simulink model "PVRobusMPC_final"  (R2018a)
settings: Solver=ode2  StartTime=0.0  StopTime=43200  FixedStep=1  RelTol=1e-3  EnableMultiTasking=on
InitFcn:
  | load PV_model_data
StopFcn:
  | save results Lambda_UV01 T_PV_Reference Tm_f01 Pout01 Tamb Time
  | clear all
  | load results
  | figure
  | subplot(3,1,1)
  | plot(Time./3600,T_PV_Reference,Time./3600,Tm_f01)
  | legend('PV Temperature Reference','PV Temperature')
  | title('MPC Tracking')
  | ylim([350 380])
  | subplot(3,1,2)
  | plot(Time./3600,Lambda_UV01)
  | ylim([250 450])
  | legend('\lambda_U_V')
  | subplot(3,1,3)
  | plot(Time./3600,Pout01)
  | legend('PV Power')
  | xlabel('Time [hours]')
  | ylabel('Watt')
values from neighbouring files (symbols this model uses):
  Global_tilt_Irr_2_2_12_13_5 = [0.000279 0.000786 0.00115 0.00401 0.0047 0.0102 0.011 0.0195 0.0266 0.0299 0.0338 0.0682 ... (2802 elements, 1401x2)]    [PV_model_data.mat]
  Total_light_absorption_in_polystyren = [0.0148235487596 0.0159326919994 0.0170383922491 0.0181406655151 0.0192395277052 0.0203349946285 0.0214270819969 0.0225158054254 0.0236011804327 0.0246832224425 0.0257619467839 0.0264640052027 ... (1151 elements, 1151x1)]    [PV_model_data.mat]
  Total_light_absorption_in_PV_cell_acrylic = [0.0222539070262 0.0239185757929 0.0255780524095 0.0272323791236 0.0288816001883 0.030525761736 0.0321649116541 0.0337990994657 0.0354283762117 0.0370527943369 0.0386724075795 0.0397267002838 ... (1151 elements, 1151x1)]    [PV_model_data.mat]
libraries: mpclib x256
(part 14 of 72)

== system PVRobusMPC_final/4 x 4 x 4 PV Panel 2/4 x 4 PV Panel 8/4 PV Panel 2/PV Panel 8/Photovolatic Panel ==
  Lambda_UV : Inport
  Lambda_IR : Inport  Port=2
  Tambient : Inport  Port=3
  WS : Inport  Port=4
  PV_Cell_Model : MATLAB Function  TreatAsAtomicUnit=on
  Step Size [sec] : Constant
  Unit Delay : UnitDelay  InitialCondition=Temp_Initial  SampleTime=-1
  Tm_f [K] : Outport
  Pout [Watt] : Outport  Port=2
  Vout [Volts] : Outport  Port=3
  wires:
  WS/1 -> PV_Cell_Model/6(WS)
  Tambient/1 -> PV_Cell_Model/5(Tambient)
  PV_Cell_Model/2(QQ) -> Pout [Watt]/1
  Unit Delay/1 -> PV_Cell_Model/1(Tm_i)
  PV_Cell_Model/1(Tm_f) -> Unit Delay/1, Tm_f [K]/1
  Lambda_UV/1 -> PV_Cell_Model/2(Lambda_UV)
  Lambda_IR/1 -> PV_Cell_Model/3(Lambda_IR)
  Step Size [sec]/1 -> PV_Cell_Model/4(Time)
  PV_Cell_Model/3(VL) -> Vout [Volts]/1

== system PVRobusMPC_final/4 x 4 x 4 PV Panel 2/4 x 4 PV Panel 8/4 PV Panel 3/PV Panel 5/PV MPC ==
  Tm_f : Inport
  Tambient : Inport  Port=2
  Fcn : Fcn  Expr=0.916 *u(1)+79
  MPC Controller : mpclib/MPC Controller  SCDEnableBlockLinearizationSpecification=on  mpcobj=mpc1  is_multiple=0  enable_value=0  return_u0=off  updateMPCinCallerWorkspace=on  ref_from_ws=off  ref_signal_name=[]  ref_preview=off  md_from_ws=off  md_signal_name=[]  md_preview=off  from_project=off  project_file=MPCtask.mat  md_inport=off  mv_inport=off  cost_outport=off  return_sequence=off  return_qpstatus=off  return_state=off  state_inport=off  lims_inport=off  cc_inport=off  ywt_inport=off  is_designfromscratch=0  uwt_inport=off  duwt_inport=off  rhoeps_inport=off  uref_inport=off  n_ts=10  n_p=10  n_mv=1  n_md=1  n_ud=0  n_mo=1  n_uo=0  BlockDataType=double  SampleTimeInherited=off  switch_inport=off
  Rate Transition1 : RateTransition  OutPortSampleTime=1
  Rate Transition2 : RateTransition  OutPortSampleTime=10
  Rate Transition3 : RateTransition  OutPortSampleTime=10
  Sum1 : Sum  Inputs=|+-
  Sum2 : Sum  Inputs=|+-
  Sum6 : Sum  Inputs=|++
  Time1 : Constant  Value=372.8
  Time3 : Constant  Value=372.8
  Time8 : Constant  Value=300
  Unit Delay2 : UnitDelay  InitialCondition=380  SampleTime=-1
  Lambda_UV : Outport
  wires:
  Unit Delay2/1 -> Sum1/1
  Time8/1 -> Sum6/2
  MPC Controller/1 -> Rate Transition1/1
  Rate Transition1/1 -> Sum6/1
  Time1/1 -> Sum2/2
  Fcn/1 -> Sum2/1
  Tambient/1 -> Fcn/1
  Sum2/1 -> Rate Transition2/1
  Sum1/1 -> Rate Transition3/1
  Rate Transition3/1 -> MPC Controller/1
  Rate Transition2/1 -> MPC Controller/2
  Sum6/1 -> Lambda_UV/1
  Time3/1 -> Sum1/2
  Tm_f/1 -> Unit Delay2/1

== system PVRobusMPC_final/4 x 4 x 4 PV Panel 2/4 x 4 PV Panel 8/4 PV Panel 3/PV Panel 5/Photovolatic Panel ==
  Lambda_UV : Inport
  Lambda_IR : Inport  Port=2
  Tambient : Inport  Port=3
  WS : Inport  Port=4
  PV_Cell_Model : MATLAB Function  TreatAsAtomicUnit=on
  Step Size [sec] : Constant
  Unit Delay : UnitDelay  InitialCondition=Temp_Initial  SampleTime=-1
  Tm_f [K] : Outport
  Pout [Watt] : Outport  Port=2
  Vout [Volts] : Outport  Port=3
  wires:
  WS/1 -> PV_Cell_Model/6(WS)
  Tambient/1 -> PV_Cell_Model/5(Tambient)
  PV_Cell_Model/2(QQ) -> Pout [Watt]/1
  Unit Delay/1 -> PV_Cell_Model/1(Tm_i)
  PV_Cell_Model/1(Tm_f) -> Unit Delay/1, Tm_f [K]/1
  Lambda_UV/1 -> PV_Cell_Model/2(Lambda_UV)
  Lambda_IR/1 -> PV_Cell_Model/3(Lambda_IR)
  Step Size [sec]/1 -> PV_Cell_Model/4(Time)
  PV_Cell_Model/3(VL) -> Vout [Volts]/1

== system PVRobusMPC_final/4 x 4 x 4 PV Panel 2/4 x 4 PV Panel 8/4 PV Panel 3/PV Panel 6/PV MPC ==
  Tm_f : Inport
  Tambient : Inport  Port=2
  Fcn : Fcn  Expr=0.916 *u(1)+79
  MPC Controller : mpclib/MPC Controller  SCDEnableBlockLinearizationSpecification=on  mpcobj=mpc1  is_multiple=0  enable_value=0  return_u0=off  updateMPCinCallerWorkspace=on  ref_from_ws=off  ref_signal_name=[]  ref_preview=off  md_from_ws=off  md_signal_name=[]  md_preview=off  from_project=off  project_file=MPCtask.mat  md_inport=off  mv_inport=off  cost_outport=off  return_sequence=off  return_qpstatus=off  return_state=off  state_inport=off  lims_inport=off  cc_inport=off  ywt_inport=off  is_designfromscratch=0  uwt_inport=off  duwt_inport=off  rhoeps_inport=off  uref_inport=off  n_ts=10  n_p=10  n_mv=1  n_md=1  n_ud=0  n_mo=1  n_uo=0  BlockDataType=double  SampleTimeInherited=off  switch_inport=off
  Rate Transition1 : RateTransition  OutPortSampleTime=1
  Rate Transition2 : RateTransition  OutPortSampleTime=10
  Rate Transition3 : RateTransition  OutPortSampleTime=10
  Sum1 : Sum  Inputs=|+-
  Sum2 : Sum  Inputs=|+-
  Sum6 : Sum  Inputs=|++
  Time1 : Constant  Value=372.8
  Time3 : Constant  Value=372.8
  Time8 : Constant  Value=300
  Unit Delay2 : UnitDelay  InitialCondition=380  SampleTime=-1
  Lambda_UV : Outport
  wires:
  Tm_f/1 -> Unit Delay2/1
  Time3/1 -> Sum1/2
  Sum6/1 -> Lambda_UV/1
  Rate Transition2/1 -> MPC Controller/2
  Rate Transition3/1 -> MPC Controller/1
  Sum1/1 -> Rate Transition3/1
  Sum2/1 -> Rate Transition2/1
  Tambient/1 -> Fcn/1
  Fcn/1 -> Sum2/1
  Time1/1 -> Sum2/2
  Rate Transition1/1 -> Sum6/1
  MPC Controller/1 -> Rate Transition1/1
  Time8/1 -> Sum6/2
  Unit Delay2/1 -> Sum1/1

== system PVRobusMPC_final/4 x 4 x 4 PV Panel 2/4 x 4 PV Panel 8/4 PV Panel 3/PV Panel 6/Photovolatic Panel ==
  Lambda_UV : Inport
  Lambda_IR : Inport  Port=2
  Tambient : Inport  Port=3
  WS : Inport  Port=4
  PV_Cell_Model : MATLAB Function  TreatAsAtomicUnit=on
  Step Size [sec] : Constant
  Unit Delay : UnitDelay  InitialCondition=Temp_Initial  SampleTime=-1
  Tm_f [K] : Outport
  Pout [Watt] : Outport  Port=2
  Vout [Volts] : Outport  Port=3
  wires:
  PV_Cell_Model/3(VL) -> Vout [Volts]/1
  Step Size [sec]/1 -> PV_Cell_Model/4(Time)
  Lambda_IR/1 -> PV_Cell_Model/3(Lambda_IR)
  Lambda_UV/1 -> PV_Cell_Model/2(Lambda_UV)
  PV_Cell_Model/1(Tm_f) -> Tm_f [K]/1, Unit Delay/1
  Unit Delay/1 -> PV_Cell_Model/1(Tm_i)
  PV_Cell_Model/2(QQ) -> Pout [Watt]/1
  Tambient/1 -> PV_Cell_Model/5(Tambient)
  WS/1 -> PV_Cell_Model/6(WS)

== system PVRobusMPC_final/4 x 4 x 4 PV Panel 2/4 x 4 PV Panel 8/4 PV Panel 3/PV Panel 7/PV MPC ==
  Tm_f : Inport
  Tambient : Inport  Port=2
  Fcn : Fcn  Expr=0.916 *u(1)+79
  MPC Controller : mpclib/MPC Controller  SCDEnableBlockLinearizationSpecification=on  mpcobj=mpc1  is_multiple=0  enable_value=0  return_u0=off  updateMPCinCallerWorkspace=on  ref_from_ws=off  ref_signal_name=[]  ref_preview=off  md_from_ws=off  md_signal_name=[]  md_preview=off  from_project=off  project_file=MPCtask.mat  md_inport=off  mv_inport=off  cost_outport=off  return_sequence=off  return_qpstatus=off  return_state=off  state_inport=off  lims_inport=off  cc_inport=off  ywt_inport=off  is_designfromscratch=0  uwt_inport=off  duwt_inport=off  rhoeps_inport=off  uref_inport=off  n_ts=10  n_p=10  n_mv=1  n_md=1  n_ud=0  n_mo=1  n_uo=0  BlockDataType=double  SampleTimeInherited=off  switch_inport=off
  Rate Transition1 : RateTransition  OutPortSampleTime=1
  Rate Transition2 : RateTransition  OutPortSampleTime=10
  Rate Transition3 : RateTransition  OutPortSampleTime=10
  Sum1 : Sum  Inputs=|+-
  Sum2 : Sum  Inputs=|+-
  Sum6 : Sum  Inputs=|++
  Time1 : Constant  Value=372.8
  Time3 : Constant  Value=372.8
  Time8 : Constant  Value=300
  Unit Delay2 : UnitDelay  InitialCondition=380  SampleTime=-1
  Lambda_UV : Outport
  wires:
  Unit Delay2/1 -> Sum1/1
  Time8/1 -> Sum6/2
  MPC Controller/1 -> Rate Transition1/1
  Rate Transition1/1 -> Sum6/1
  Time1/1 -> Sum2/2
  Fcn/1 -> Sum2/1
  Tambient/1 -> Fcn/1
  Sum2/1 -> Rate Transition2/1
  Sum1/1 -> Rate Transition3/1
  Rate Transition3/1 -> MPC Controller/1
  Rate Transition2/1 -> MPC Controller/2
  Sum6/1 -> Lambda_UV/1
  Time3/1 -> Sum1/2
  Tm_f/1 -> Unit Delay2/1

== system PVRobusMPC_final/4 x 4 x 4 PV Panel 2/4 x 4 PV Panel 8/4 PV Panel 3/PV Panel 7/Photovolatic Panel ==
  Lambda_UV : Inport
  Lambda_IR : Inport  Port=2
  Tambient : Inport  Port=3
  WS : Inport  Port=4
  PV_Cell_Model : MATLAB Function  TreatAsAtomicUnit=on
  Step Size [sec] : Constant
  Unit Delay : UnitDelay  InitialCondition=Temp_Initial  SampleTime=-1
  Tm_f [K] : Outport
  Pout [Watt] : Outport  Port=2
  Vout [Volts] : Outport  Port=3
  wires:
  WS/1 -> PV_Cell_Model/6(WS)
  Tambient/1 -> PV_Cell_Model/5(Tambient)
  PV_Cell_Model/2(QQ) -> Pout [Watt]/1
  Unit Delay/1 -> PV_Cell_Model/1(Tm_i)
  PV_Cell_Model/1(Tm_f) -> Unit Delay/1, Tm_f [K]/1
  Lambda_UV/1 -> PV_Cell_Model/2(Lambda_UV)
  Lambda_IR/1 -> PV_Cell_Model/3(Lambda_IR)
  Step Size [sec]/1 -> PV_Cell_Model/4(Time)
  PV_Cell_Model/3(VL) -> Vout [Volts]/1

== system PVRobusMPC_final/4 x 4 x 4 PV Panel 2/4 x 4 PV Panel 8/4 PV Panel 3/PV Panel 8/PV MPC ==
  Tm_f : Inport
  Tambient : Inport  Port=2
  Fcn : Fcn  Expr=0.916 *u(1)+79
  MPC Controller : mpclib/MPC Controller  SCDEnableBlockLinearizationSpecification=on  mpcobj=mpc1  is_multiple=0  enable_value=0  return_u0=off  updateMPCinCallerWorkspace=on  ref_from_ws=off  ref_signal_name=[]  ref_preview=off  md_from_ws=off  md_signal_name=[]  md_preview=off  from_project=off  project_file=MPCtask.mat  md_inport=off  mv_inport=off  cost_outport=off  return_sequence=off  return_qpstatus=off  return_state=off  state_inport=off  lims_inport=off  cc_inport=off  ywt_inport=off  is_designfromscratch=0  uwt_inport=off  duwt_inport=off  rhoeps_inport=off  uref_inport=off  n_ts=10  n_p=10  n_mv=1  n_md=1  n_ud=0  n_mo=1  n_uo=0  BlockDataType=double  SampleTimeInherited=off  switch_inport=off
  Rate Transition1 : RateTransition  OutPortSampleTime=1
  Rate Transition2 : RateTransition  OutPortSampleTime=10
  Rate Transition3 : RateTransition  OutPortSampleTime=10
  Sum1 : Sum  Inputs=|+-
  Sum2 : Sum  Inputs=|+-
  Sum6 : Sum  Inputs=|++
  Time1 : Constant  Value=372.8
  Time3 : Constant  Value=372.8
  Time8 : Constant  Value=300
  Unit Delay2 : UnitDelay  InitialCondition=380  SampleTime=-1
  Lambda_UV : Outport
  wires:
  Tm_f/1 -> Unit Delay2/1
  Time3/1 -> Sum1/2
  Sum6/1 -> Lambda_UV/1
  Rate Transition2/1 -> MPC Controller/2
  Rate Transition3/1 -> MPC Controller/1
  Sum1/1 -> Rate Transition3/1
  Sum2/1 -> Rate Transition2/1
  Tambient/1 -> Fcn/1
  Fcn/1 -> Sum2/1
  Time1/1 -> Sum2/2
  Rate Transition1/1 -> Sum6/1
  MPC Controller/1 -> Rate Transition1/1
  Time8/1 -> Sum6/2
  Unit Delay2/1 -> Sum1/1

== system PVRobusMPC_final/4 x 4 x 4 PV Panel 2/4 x 4 PV Panel 8/4 PV Panel 3/PV Panel 8/Photovolatic Panel ==
  Lambda_UV : Inport
  Lambda_IR : Inport  Port=2
  Tambient : Inport  Port=3
  WS : Inport  Port=4
  PV_Cell_Model : MATLAB Function  TreatAsAtomicUnit=on
  Step Size [sec] : Constant
  Unit Delay : UnitDelay  InitialCondition=Temp_Initial  SampleTime=-1
  Tm_f [K] : Outport
  Pout [Watt] : Outport  Port=2
  Vout [Volts] : Outport  Port=3
  wires:
  PV_Cell_Model/3(VL) -> Vout [Volts]/1
  Step Size [sec]/1 -> PV_Cell_Model/4(Time)
  Lambda_IR/1 -> PV_Cell_Model/3(Lambda_IR)
  Lambda_UV/1 -> PV_Cell_Model/2(Lambda_UV)
  PV_Cell_Model/1(Tm_f) -> Tm_f [K]/1, Unit Delay/1
  Unit Delay/1 -> PV_Cell_Model/1(Tm_i)
  PV_Cell_Model/2(QQ) -> Pout [Watt]/1
  Tambient/1 -> PV_Cell_Model/5(Tambient)
  WS/1 -> PV_Cell_Model/6(WS)

== system PVRobusMPC_final/4 x 4 x 4 PV Panel 2/4 x 4 PV Panel 8/4 PV Panel 4/PV Panel 5/PV MPC ==
  Tm_f : Inport
  Tambient : Inport  Port=2
  Fcn : Fcn  Expr=0.916 *u(1)+79
  MPC Controller : mpclib/MPC Controller  SCDEnableBlockLinearizationSpecification=on  mpcobj=mpc1  is_multiple=0  enable_value=0  return_u0=off  updateMPCinCallerWorkspace=on  ref_from_ws=off  ref_signal_name=[]  ref_preview=off  md_from_ws=off  md_signal_name=[]  md_preview=off  from_project=off  project_file=MPCtask.mat  md_inport=off  mv_inport=off  cost_outport=off  return_sequence=off  return_qpstatus=off  return_state=off  state_inport=off  lims_inport=off  cc_inport=off  ywt_inport=off  is_designfromscratch=0  uwt_inport=off  duwt_inport=off  rhoeps_inport=off  uref_inport=off  n_ts=10  n_p=10  n_mv=1  n_md=1  n_ud=0  n_mo=1  n_uo=0  BlockDataType=double  SampleTimeInherited=off  switch_inport=off
  Rate Transition1 : RateTransition  OutPortSampleTime=1
  Rate Transition2 : RateTransition  OutPortSampleTime=10
  Rate Transition3 : RateTransition  OutPortSampleTime=10
  Sum1 : Sum  Inputs=|+-
  Sum2 : Sum  Inputs=|+-
  Sum6 : Sum  Inputs=|++
  Time1 : Constant  Value=372.8
  Time3 : Constant  Value=372.8
  Time8 : Constant  Value=300
  Unit Delay2 : UnitDelay  InitialCondition=380  SampleTime=-1
  Lambda_UV : Outport
  wires:
  Tm_f/1 -> Unit Delay2/1
  Time3/1 -> Sum1/2
  Sum6/1 -> Lambda_UV/1
  Rate Transition2/1 -> MPC Controller/2
  Rate Transition3/1 -> MPC Controller/1
  Sum1/1 -> Rate Transition3/1
  Sum2/1 -> Rate Transition2/1
  Tambient/1 -> Fcn/1
  Fcn/1 -> Sum2/1
  Time1/1 -> Sum2/2
  Rate Transition1/1 -> Sum6/1
  MPC Controller/1 -> Rate Transition1/1
  Time8/1 -> Sum6/2
  Unit Delay2/1 -> Sum1/1

== system PVRobusMPC_final/4 x 4 x 4 PV Panel 2/4 x 4 PV Panel 8/4 PV Panel 4/PV Panel 5/Photovolatic Panel ==
  Lambda_UV : Inport
  Lambda_IR : Inport  Port=2
  Tambient : Inport  Port=3
  WS : Inport  Port=4
  PV_Cell_Model : MATLAB Function  TreatAsAtomicUnit=on
  Step Size [sec] : Constant
  Unit Delay : UnitDelay  InitialCondition=Temp_Initial  SampleTime=-1
  Tm_f [K] : Outport
  Pout [Watt] : Outport  Port=2
  Vout [Volts] : Outport  Port=3
  wires:
  PV_Cell_Model/3(VL) -> Vout [Volts]/1
  Step Size [sec]/1 -> PV_Cell_Model/4(Time)
  Lambda_IR/1 -> PV_Cell_Model/3(Lambda_IR)
  Lambda_UV/1 -> PV_Cell_Model/2(Lambda_UV)
  PV_Cell_Model/1(Tm_f) -> Tm_f [K]/1, Unit Delay/1
  Unit Delay/1 -> PV_Cell_Model/1(Tm_i)
  PV_Cell_Model/2(QQ) -> Pout [Watt]/1
  Tambient/1 -> PV_Cell_Model/5(Tambient)
  WS/1 -> PV_Cell_Model/6(WS)

== system PVRobusMPC_final/4 x 4 x 4 PV Panel 2/4 x 4 PV Panel 8/4 PV Panel 4/PV Panel 6/PV MPC ==
  Tm_f : Inport
  Tambient : Inport  Port=2
  Fcn : Fcn  Expr=0.916 *u(1)+79
  MPC Controller : mpclib/MPC Controller  SCDEnableBlockLinearizationSpecification=on  mpcobj=mpc1  is_multiple=0  enable_value=0  return_u0=off  updateMPCinCallerWorkspace=on  ref_from_ws=off  ref_signal_name=[]  ref_preview=off  md_from_ws=off  md_signal_name=[]  md_preview=off  from_project=off  project_file=MPCtask.mat  md_inport=off  mv_inport=off  cost_outport=off  return_sequence=off  return_qpstatus=off  return_state=off  state_inport=off  lims_inport=off  cc_inport=off  ywt_inport=off  is_designfromscratch=0  uwt_inport=off  duwt_inport=off  rhoeps_inport=off  uref_inport=off  n_ts=10  n_p=10  n_mv=1  n_md=1  n_ud=0  n_mo=1  n_uo=0  BlockDataType=double  SampleTimeInherited=off  switch_inport=off
  Rate Transition1 : RateTransition  OutPortSampleTime=1
  Rate Transition2 : RateTransition  OutPortSampleTime=10
  Rate Transition3 : RateTransition  OutPortSampleTime=10
  Sum1 : Sum  Inputs=|+-
  Sum2 : Sum  Inputs=|+-
  Sum6 : Sum  Inputs=|++
  Time1 : Constant  Value=372.8
  Time3 : Constant  Value=372.8
  Time8 : Constant  Value=300
  Unit Delay2 : UnitDelay  InitialCondition=380  SampleTime=-1
  Lambda_UV : Outport
  wires:
  Unit Delay2/1 -> Sum1/1
  Time8/1 -> Sum6/2
  MPC Controller/1 -> Rate Transition1/1
  Rate Transition1/1 -> Sum6/1
  Time1/1 -> Sum2/2
  Fcn/1 -> Sum2/1
  Tambient/1 -> Fcn/1
  Sum2/1 -> Rate Transition2/1
  Sum1/1 -> Rate Transition3/1
  Rate Transition3/1 -> MPC Controller/1
  Rate Transition2/1 -> MPC Controller/2
  Sum6/1 -> Lambda_UV/1
  Time3/1 -> Sum1/2
  Tm_f/1 -> Unit Delay2/1

== system PVRobusMPC_final/4 x 4 x 4 PV Panel 2/4 x 4 PV Panel 8/4 PV Panel 4/PV Panel 6/Photovolatic Panel ==
  Lambda_UV : Inport
  Lambda_IR : Inport  Port=2
  Tambient : Inport  Port=3
  WS : Inport  Port=4
  PV_Cell_Model : MATLAB Function  TreatAsAtomicUnit=on
  Step Size [sec] : Constant
  Unit Delay : UnitDelay  InitialCondition=Temp_Initial  SampleTime=-1
  Tm_f [K] : Outport
  Pout [Watt] : Outport  Port=2
  Vout [Volts] : Outport  Port=3
  wires:
  WS/1 -> PV_Cell_Model/6(WS)
  Tambient/1 -> PV_Cell_Model/5(Tambient)
  PV_Cell_Model/2(QQ) -> Pout [Watt]/1
  Unit Delay/1 -> PV_Cell_Model/1(Tm_i)
  PV_Cell_Model/1(Tm_f) -> Unit Delay/1, Tm_f [K]/1
  Lambda_UV/1 -> PV_Cell_Model/2(Lambda_UV)
  Lambda_IR/1 -> PV_Cell_Model/3(Lambda_IR)
  Step Size [sec]/1 -> PV_Cell_Model/4(Time)
  PV_Cell_Model/3(VL) -> Vout [Volts]/1

== system PVRobusMPC_final/4 x 4 x 4 PV Panel 2/4 x 4 PV Panel 8/4 PV Panel 4/PV Panel 7/PV MPC ==
  Tm_f : Inport
  Tambient : Inport  Port=2
  Fcn : Fcn  Expr=0.916 *u(1)+79
  MPC Controller : mpclib/MPC Controller  SCDEnableBlockLinearizationSpecification=on  mpcobj=mpc1  is_multiple=0  enable_value=0  return_u0=off  updateMPCinCallerWorkspace=on  ref_from_ws=off  ref_signal_name=[]  ref_preview=off  md_from_ws=off  md_signal_name=[]  md_preview=off  from_project=off  project_file=MPCtask.mat  md_inport=off  mv_inport=off  cost_outport=off  return_sequence=off  return_qpstatus=off  return_state=off  state_inport=off  lims_inport=off  cc_inport=off  ywt_inport=off  is_designfromscratch=0  uwt_inport=off  duwt_inport=off  rhoeps_inport=off  uref_inport=off  n_ts=10  n_p=10  n_mv=1  n_md=1  n_ud=0  n_mo=1  n_uo=0  BlockDataType=double  SampleTimeInherited=off  switch_inport=off
  Rate Transition1 : RateTransition  OutPortSampleTime=1
  Rate Transition2 : RateTransition  OutPortSampleTime=10
  Rate Transition3 : RateTransition  OutPortSampleTime=10
  Sum1 : Sum  Inputs=|+-
  Sum2 : Sum  Inputs=|+-
  Sum6 : Sum  Inputs=|++
  Time1 : Constant  Value=372.8
  Time3 : Constant  Value=372.8
  Time8 : Constant  Value=300
  Unit Delay2 : UnitDelay  InitialCondition=380  SampleTime=-1
  Lambda_UV : Outport
  wires:
  Tm_f/1 -> Unit Delay2/1
  Time3/1 -> Sum1/2
  Sum6/1 -> Lambda_UV/1
  Rate Transition2/1 -> MPC Controller/2
  Rate Transition3/1 -> MPC Controller/1
  Sum1/1 -> Rate Transition3/1
  Sum2/1 -> Rate Transition2/1
  Tambient/1 -> Fcn/1
  Fcn/1 -> Sum2/1
  Time1/1 -> Sum2/2
  Rate Transition1/1 -> Sum6/1
  MPC Controller/1 -> Rate Transition1/1
  Time8/1 -> Sum6/2
  Unit Delay2/1 -> Sum1/1

== system PVRobusMPC_final/4 x 4 x 4 PV Panel 2/4 x 4 PV Panel 8/4 PV Panel 4/PV Panel 7/Photovolatic Panel ==
  Lambda_UV : Inport
  Lambda_IR : Inport  Port=2
  Tambient : Inport  Port=3
  WS : Inport  Port=4
  PV_Cell_Model : MATLAB Function  TreatAsAtomicUnit=on
  Step Size [sec] : Constant
  Unit Delay : UnitDelay  InitialCondition=Temp_Initial  SampleTime=-1
  Tm_f [K] : Outport
  Pout [Watt] : Outport  Port=2
  Vout [Volts] : Outport  Port=3
  wires:
  PV_Cell_Model/3(VL) -> Vout [Volts]/1
  Step Size [sec]/1 -> PV_Cell_Model/4(Time)
  Lambda_IR/1 -> PV_Cell_Model/3(Lambda_IR)
  Lambda_UV/1 -> PV_Cell_Model/2(Lambda_UV)
  PV_Cell_Model/1(Tm_f) -> Tm_f [K]/1, Unit Delay/1
  Unit Delay/1 -> PV_Cell_Model/1(Tm_i)
  PV_Cell_Model/2(QQ) -> Pout [Watt]/1
  Tambient/1 -> PV_Cell_Model/5(Tambient)
  WS/1 -> PV_Cell_Model/6(WS)

== system PVRobusMPC_final/4 x 4 x 4 PV Panel 2/4 x 4 PV Panel 8/4 PV Panel 4/PV Panel 8/PV MPC ==
  Tm_f : Inport
  Tambient : Inport  Port=2
  Fcn : Fcn  Expr=0.916 *u(1)+79
  MPC Controller : mpclib/MPC Controller  SCDEnableBlockLinearizationSpecification=on  mpcobj=mpc1  is_multiple=0  enable_value=0  return_u0=off  updateMPCinCallerWorkspace=on  ref_from_ws=off  ref_signal_name=[]  ref_preview=off  md_from_ws=off  md_signal_name=[]  md_preview=off  from_project=off  project_file=MPCtask.mat  md_inport=off  mv_inport=off  cost_outport=off  return_sequence=off  return_qpstatus=off  return_state=off  state_inport=off  lims_inport=off  cc_inport=off  ywt_inport=off  is_designfromscratch=0  uwt_inport=off  duwt_inport=off  rhoeps_inport=off  uref_inport=off  n_ts=10  n_p=10  n_mv=1  n_md=1  n_ud=0  n_mo=1  n_uo=0  BlockDataType=double  SampleTimeInherited=off  switch_inport=off
  Rate Transition1 : RateTransition  OutPortSampleTime=1
  Rate Transition2 : RateTransition  OutPortSampleTime=10
  Rate Transition3 : RateTransition  OutPortSampleTime=10
  Sum1 : Sum  Inputs=|+-
  Sum2 : Sum  Inputs=|+-
  Sum6 : Sum  Inputs=|++
  Time1 : Constant  Value=372.8
  Time3 : Constant  Value=372.8
  Time8 : Constant  Value=300
  Unit Delay2 : UnitDelay  InitialCondition=380  SampleTime=-1
  Lambda_UV : Outport
  wires:
  Unit Delay2/1 -> Sum1/1
  Time8/1 -> Sum6/2
  MPC Controller/1 -> Rate Transition1/1
  Rate Transition1/1 -> Sum6/1
  Time1/1 -> Sum2/2
  Fcn/1 -> Sum2/1
  Tambient/1 -> Fcn/1
  Sum2/1 -> Rate Transition2/1
  Sum1/1 -> Rate Transition3/1
  Rate Transition3/1 -> MPC Controller/1
  Rate Transition2/1 -> MPC Controller/2
  Sum6/1 -> Lambda_UV/1
  Time3/1 -> Sum1/2
  Tm_f/1 -> Unit Delay2/1

== system PVRobusMPC_final/4 x 4 x 4 PV Panel 2/4 x 4 PV Panel 8/4 PV Panel 4/PV Panel 8/Photovolatic Panel ==
  Lambda_UV : Inport
  Lambda_IR : Inport  Port=2
  Tambient : Inport  Port=3
  WS : Inport  Port=4
  PV_Cell_Model : MATLAB Function  TreatAsAtomicUnit=on
  Step Size [sec] : Constant
  Unit Delay : UnitDelay  InitialCondition=Temp_Initial  SampleTime=-1
  Tm_f [K] : Outport
  Pout [Watt] : Outport  Port=2
  Vout [Volts] : Outport  Port=3
  wires:
  WS/1 -> PV_Cell_Model/6(WS)
  Tambient/1 -> PV_Cell_Model/5(Tambient)
  PV_Cell_Model/2(QQ) -> Pout [Watt]/1
  Unit Delay/1 -> PV_Cell_Model/1(Tm_i)
  PV_Cell_Model/1(Tm_f) -> Unit Delay/1, Tm_f [K]/1
  Lambda_UV/1 -> PV_Cell_Model/2(Lambda_UV)
  Lambda_IR/1 -> PV_Cell_Model/3(Lambda_IR)
  Step Size [sec]/1 -> PV_Cell_Model/4(Time)
  PV_Cell_Model/3(VL) -> Vout [Volts]/1

== system PVRobusMPC_final/4 x 4 x 4 PV Panel 3/4 x 4 PV Panel 5/4 PV Panel 1/PV Panel 1/PV MPC ==
  Tm_f : Inport
  Tambient : Inport  Port=2
  Fcn : Fcn  Expr=0.916 *u(1)+79
  MPC Controller : mpclib/MPC Controller  SCDEnableBlockLinearizationSpecification=on  mpcobj=mpc1  is_multiple=0  enable_value=0  return_u0=off  updateMPCinCallerWorkspace=on  ref_from_ws=off  ref_signal_name=[]  ref_preview=off  md_from_ws=off  md_signal_name=[]  md_preview=off  from_project=off  project_file=MPCtask.mat  md_inport=off  mv_inport=off  cost_outport=off  return_sequence=off  return_qpstatus=off  return_state=off  state_inport=off  lims_inport=off  cc_inport=off  ywt_inport=off  is_designfromscratch=0  uwt_inport=off  duwt_inport=off  rhoeps_inport=off  uref_inport=off  n_ts=10  n_p=10  n_mv=1  n_md=1  n_ud=0  n_mo=1  n_uo=0  BlockDataType=double  SampleTimeInherited=off  switch_inport=off
  Rate Transition1 : RateTransition  OutPortSampleTime=1
  Rate Transition2 : RateTransition  OutPortSampleTime=10
  Rate Transition3 : RateTransition  OutPortSampleTime=10
  Sum1 : Sum  Inputs=|+-
  Sum2 : Sum  Inputs=|+-
  Sum6 : Sum  Inputs=|++
  Time1 : Constant  Value=372.8
  Time3 : Constant  Value=372.8
  Time8 : Constant  Value=300
  Unit Delay2 : UnitDelay  InitialCondition=380  SampleTime=-1
  Lambda_UV : Outport
  wires:
  Tm_f/1 -> Unit Delay2/1
  Time3/1 -> Sum1/2
  Sum6/1 -> Lambda_UV/1
  Rate Transition2/1 -> MPC Controller/2
  Rate Transition3/1 -> MPC Controller/1
  Sum1/1 -> Rate Transition3/1
  Sum2/1 -> Rate Transition2/1
  Tambient/1 -> Fcn/1
  Fcn/1 -> Sum2/1
  Time1/1 -> Sum2/2
  Rate Transition1/1 -> Sum6/1
  MPC Controller/1 -> Rate Transition1/1
  Time8/1 -> Sum6/2
  Unit Delay2/1 -> Sum1/1

== system PVRobusMPC_final/4 x 4 x 4 PV Panel 3/4 x 4 PV Panel 5/4 PV Panel 1/PV Panel 1/Photovolatic Panel ==
  Lambda_UV : Inport
  Lambda_IR : Inport  Port=2
  Tambient : Inport  Port=3
  WS : Inport  Port=4
  PV_Cell_Model : MATLAB Function  TreatAsAtomicUnit=on
  Step Size [sec] : Constant
  Unit Delay : UnitDelay  InitialCondition=Temp_Initial  SampleTime=-1
  Tm_f [K] : Outport
  Pout [Watt] : Outport  Port=2
  Vout [Volts] : Outport  Port=3
  wires:
  PV_Cell_Model/3(VL) -> Vout [Volts]/1
  Step Size [sec]/1 -> PV_Cell_Model/4(Time)
  Lambda_IR/1 -> PV_Cell_Model/3(Lambda_IR)
  Lambda_UV/1 -> PV_Cell_Model/2(Lambda_UV)
  PV_Cell_Model/1(Tm_f) -> Tm_f [K]/1, Unit Delay/1
  Unit Delay/1 -> PV_Cell_Model/1(Tm_i)
  PV_Cell_Model/2(QQ) -> Pout [Watt]/1
  Tambient/1 -> PV_Cell_Model/5(Tambient)
  WS/1 -> PV_Cell_Model/6(WS)

== system PVRobusMPC_final/4 x 4 x 4 PV Panel 3/4 x 4 PV Panel 5/4 PV Panel 1/PV Panel 2/PV MPC ==
  Tm_f : Inport
  Tambient : Inport  Port=2
  Fcn : Fcn  Expr=0.916 *u(1)+79
  MPC Controller : mpclib/MPC Controller  SCDEnableBlockLinearizationSpecification=on  mpcobj=mpc1  is_multiple=0  enable_value=0  return_u0=off  updateMPCinCallerWorkspace=on  ref_from_ws=off  ref_signal_name=[]  ref_preview=off  md_from_ws=off  md_signal_name=[]  md_preview=off  from_project=off  project_file=MPCtask.mat  md_inport=off  mv_inport=off  cost_outport=off  return_sequence=off  return_qpstatus=off  return_state=off  state_inport=off  lims_inport=off  cc_inport=off  ywt_inport=off  is_designfromscratch=0  uwt_inport=off  duwt_inport=off  rhoeps_inport=off  uref_inport=off  n_ts=10  n_p=10  n_mv=1  n_md=1  n_ud=0  n_mo=1  n_uo=0  BlockDataType=double  SampleTimeInherited=off  switch_inport=off
  Rate Transition1 : RateTransition  OutPortSampleTime=1
  Rate Transition2 : RateTransition  OutPortSampleTime=10
  Rate Transition3 : RateTransition  OutPortSampleTime=10
  Sum1 : Sum  Inputs=|+-
  Sum2 : Sum  Inputs=|+-
  Sum6 : Sum  Inputs=|++
  Time1 : Constant  Value=372.8
  Time3 : Constant  Value=372.8
  Time8 : Constant  Value=300
  Unit Delay2 : UnitDelay  InitialCondition=380  SampleTime=-1
  Lambda_UV : Outport
  wires:
  Unit Delay2/1 -> Sum1/1
  Time8/1 -> Sum6/2
  MPC Controller/1 -> Rate Transition1/1
  Rate Transition1/1 -> Sum6/1
  Time1/1 -> Sum2/2
  Fcn/1 -> Sum2/1
  Tambient/1 -> Fcn/1
  Sum2/1 -> Rate Transition2/1
  Sum1/1 -> Rate Transition3/1
  Rate Transition3/1 -> MPC Controller/1
  Rate Transition2/1 -> MPC Controller/2
  Sum6/1 -> Lambda_UV/1
  Time3/1 -> Sum1/2
  Tm_f/1 -> Unit Delay2/1

== system PVRobusMPC_final/4 x 4 x 4 PV Panel 3/4 x 4 PV Panel 5/4 PV Panel 1/PV Panel 2/Photovolatic Panel ==
  Lambda_UV : Inport
  Lambda_IR : Inport  Port=2
  Tambient : Inport  Port=3
  WS : Inport  Port=4
  PV_Cell_Model : MATLAB Function  TreatAsAtomicUnit=on
  Step Size [sec] : Constant
  Unit Delay : UnitDelay  InitialCondition=Temp_Initial  SampleTime=-1
  Tm_f [K] : Outport
  Pout [Watt] : Outport  Port=2
  Vout [Volts] : Outport  Port=3
  wires:
  WS/1 -> PV_Cell_Model/6(WS)
  Tambient/1 -> PV_Cell_Model/5(Tambient)
  PV_Cell_Model/2(QQ) -> Pout [Watt]/1
  Unit Delay/1 -> PV_Cell_Model/1(Tm_i)
  PV_Cell_Model/1(Tm_f) -> Unit Delay/1, Tm_f [K]/1
  Lambda_UV/1 -> PV_Cell_Model/2(Lambda_UV)
  Lambda_IR/1 -> PV_Cell_Model/3(Lambda_IR)
  Step Size [sec]/1 -> PV_Cell_Model/4(Time)
  PV_Cell_Model/3(VL) -> Vout [Volts]/1

== system PVRobusMPC_final/4 x 4 x 4 PV Panel 3/4 x 4 PV Panel 5/4 PV Panel 1/PV Panel 3/PV MPC ==
  Tm_f : Inport
  Tambient : Inport  Port=2
  Fcn : Fcn  Expr=0.916 *u(1)+79
  MPC Controller : mpclib/MPC Controller  SCDEnableBlockLinearizationSpecification=on  mpcobj=mpc1  is_multiple=0  enable_value=0  return_u0=off  updateMPCinCallerWorkspace=on  ref_from_ws=off  ref_signal_name=[]  ref_preview=off  md_from_ws=off  md_signal_name=[]  md_preview=off  from_project=off  project_file=MPCtask.mat  md_inport=off  mv_inport=off  cost_outport=off  return_sequence=off  return_qpstatus=off  return_state=off  state_inport=off  lims_inport=off  cc_inport=off  ywt_inport=off  is_designfromscratch=0  uwt_inport=off  duwt_inport=off  rhoeps_inport=off  uref_inport=off  n_ts=10  n_p=10  n_mv=1  n_md=1  n_ud=0  n_mo=1  n_uo=0  BlockDataType=double  SampleTimeInherited=off  switch_inport=off
  Rate Transition1 : RateTransition  OutPortSampleTime=1
  Rate Transition2 : RateTransition  OutPortSampleTime=10
  Rate Transition3 : RateTransition  OutPortSampleTime=10
  Sum1 : Sum  Inputs=|+-
  Sum2 : Sum  Inputs=|+-
  Sum6 : Sum  Inputs=|++
  Time1 : Constant  Value=372.8
  Time3 : Constant  Value=372.8
  Time8 : Constant  Value=300
  Unit Delay2 : UnitDelay  InitialCondition=380  SampleTime=-1
  Lambda_UV : Outport
  wires:
  Tm_f/1 -> Unit Delay2/1
  Time3/1 -> Sum1/2
  Sum6/1 -> Lambda_UV/1
  Rate Transition2/1 -> MPC Controller/2
  Rate Transition3/1 -> MPC Controller/1
  Sum1/1 -> Rate Transition3/1
  Sum2/1 -> Rate Transition2/1
  Tambient/1 -> Fcn/1
  Fcn/1 -> Sum2/1
  Time1/1 -> Sum2/2
  Rate Transition1/1 -> Sum6/1
  MPC Controller/1 -> Rate Transition1/1
  Time8/1 -> Sum6/2
  Unit Delay2/1 -> Sum1/1

== system PVRobusMPC_final/4 x 4 x 4 PV Panel 3/4 x 4 PV Panel 5/4 PV Panel 1/PV Panel 3/Photovolatic Panel ==
  Lambda_UV : Inport
  Lambda_IR : Inport  Port=2
  Tambient : Inport  Port=3
  WS : Inport  Port=4
  PV_Cell_Model : MATLAB Function  TreatAsAtomicUnit=on
  Step Size [sec] : Constant
  Unit Delay : UnitDelay  InitialCondition=Temp_Initial  SampleTime=-1
  Tm_f [K] : Outport
  Pout [Watt] : Outport  Port=2
  Vout [Volts] : Outport  Port=3
  wires:
  PV_Cell_Model/3(VL) -> Vout [Volts]/1
  Step Size [sec]/1 -> PV_Cell_Model/4(Time)
  Lambda_IR/1 -> PV_Cell_Model/3(Lambda_IR)
  Lambda_UV/1 -> PV_Cell_Model/2(Lambda_UV)
  PV_Cell_Model/1(Tm_f) -> Tm_f [K]/1, Unit Delay/1
  Unit Delay/1 -> PV_Cell_Model/1(Tm_i)
  PV_Cell_Model/2(QQ) -> Pout [Watt]/1
  Tambient/1 -> PV_Cell_Model/5(Tambient)
  WS/1 -> PV_Cell_Model/6(WS)

== system PVRobusMPC_final/4 x 4 x 4 PV Panel 3/4 x 4 PV Panel 5/4 PV Panel 1/PV Panel 4/PV MPC ==
  Tm_f : Inport
  Tambient : Inport  Port=2
  Fcn : Fcn  Expr=0.916 *u(1)+79
  MPC Controller : mpclib/MPC Controller  SCDEnableBlockLinearizationSpecification=on  mpcobj=mpc1  is_multiple=0  enable_value=0  return_u0=off  updateMPCinCallerWorkspace=on  ref_from_ws=off  ref_signal_name=[]  ref_preview=off  md_from_ws=off  md_signal_name=[]  md_preview=off  from_project=off  project_file=MPCtask.mat  md_inport=off  mv_inport=off  cost_outport=off  return_sequence=off  return_qpstatus=off  return_state=off  state_inport=off  lims_inport=off  cc_inport=off  ywt_inport=off  is_designfromscratch=0  uwt_inport=off  duwt_inport=off  rhoeps_inport=off  uref_inport=off  n_ts=10  n_p=10  n_mv=1  n_md=1  n_ud=0  n_mo=1  n_uo=0  BlockDataType=double  SampleTimeInherited=off  switch_inport=off
  Rate Transition1 : RateTransition  OutPortSampleTime=1
  Rate Transition2 : RateTransition  OutPortSampleTime=10
  Rate Transition3 : RateTransition  OutPortSampleTime=10
  Sum1 : Sum  Inputs=|+-
  Sum2 : Sum  Inputs=|+-
  Sum6 : Sum  Inputs=|++
  Time1 : Constant  Value=372.8
  Time3 : Constant  Value=372.8
  Time8 : Constant  Value=300
  Unit Delay2 : UnitDelay  InitialCondition=380  SampleTime=-1
  Lambda_UV : Outport
  wires:
  Unit Delay2/1 -> Sum1/1
  Time8/1 -> Sum6/2
  MPC Controller/1 -> Rate Transition1/1
  Rate Transition1/1 -> Sum6/1
  Time1/1 -> Sum2/2
  Fcn/1 -> Sum2/1
  Tambient/1 -> Fcn/1
  Sum2/1 -> Rate Transition2/1
  Sum1/1 -> Rate Transition3/1
  Rate Transition3/1 -> MPC Controller/1
  Rate Transition2/1 -> MPC Controller/2
  Sum6/1 -> Lambda_UV/1
  Time3/1 -> Sum1/2
  Tm_f/1 -> Unit Delay2/1

== system PVRobusMPC_final/4 x 4 x 4 PV Panel 3/4 x 4 PV Panel 5/4 PV Panel 1/PV Panel 4/Photovolatic Panel ==
  Lambda_UV : Inport
  Lambda_IR : Inport  Port=2
  Tambient : Inport  Port=3
  WS : Inport  Port=4
  PV_Cell_Model : MATLAB Function  TreatAsAtomicUnit=on
  Step Size [sec] : Constant
  Unit Delay : UnitDelay  InitialCondition=Temp_Initial  SampleTime=-1
  Tm_f [K] : Outport
  Pout [Watt] : Outport  Port=2
  Vout [Volts] : Outport  Port=3
  wires:
  WS/1 -> PV_Cell_Model/6(WS)
  Tambient/1 -> PV_Cell_Model/5(Tambient)
  PV_Cell_Model/2(QQ) -> Pout [Watt]/1
  Unit Delay/1 -> PV_Cell_Model/1(Tm_i)
  PV_Cell_Model/1(Tm_f) -> Unit Delay/1, Tm_f [K]/1
  Lambda_UV/1 -> PV_Cell_Model/2(Lambda_UV)
  Lambda_IR/1 -> PV_Cell_Model/3(Lambda_IR)
  Step Size [sec]/1 -> PV_Cell_Model/4(Time)
  PV_Cell_Model/3(VL) -> Vout [Volts]/1

== system PVRobusMPC_final/4 x 4 x 4 PV Panel 3/4 x 4 PV Panel 5/4 PV Panel 2/PV Panel 5/PV MPC ==
  Tm_f : Inport
  Tambient : Inport  Port=2
  Fcn : Fcn  Expr=0.916 *u(1)+79
  MPC Controller : mpclib/MPC Controller  SCDEnableBlockLinearizationSpecification=on  mpcobj=mpc1  is_multiple=0  enable_value=0  return_u0=off  updateMPCinCallerWorkspace=on  ref_from_ws=off  ref_signal_name=[]  ref_preview=off  md_from_ws=off  md_signal_name=[]  md_preview=off  from_project=off  project_file=MPCtask.mat  md_inport=off  mv_inport=off  cost_outport=off  return_sequence=off  return_qpstatus=off  return_state=off  state_inport=off  lims_inport=off  cc_inport=off  ywt_inport=off  is_designfromscratch=0  uwt_inport=off  duwt_inport=off  rhoeps_inport=off  uref_inport=off  n_ts=10  n_p=10  n_mv=1  n_md=1  n_ud=0  n_mo=1  n_uo=0  BlockDataType=double  SampleTimeInherited=off  switch_inport=off
  Rate Transition1 : RateTransition  OutPortSampleTime=1
  Rate Transition2 : RateTransition  OutPortSampleTime=10
  Rate Transition3 : RateTransition  OutPortSampleTime=10
  Sum1 : Sum  Inputs=|+-
  Sum2 : Sum  Inputs=|+-
  Sum6 : Sum  Inputs=|++
  Time1 : Constant  Value=372.8
  Time3 : Constant  Value=372.8
  Time8 : Constant  Value=300
  Unit Delay2 : UnitDelay  InitialCondition=380  SampleTime=-1
  Lambda_UV : Outport
  wires:
  Tm_f/1 -> Unit Delay2/1
  Time3/1 -> Sum1/2
  Sum6/1 -> Lambda_UV/1
  Rate Transition2/1 -> MPC Controller/2
  Rate Transition3/1 -> MPC Controller/1
  Sum1/1 -> Rate Transition3/1
  Sum2/1 -> Rate Transition2/1
  Tambient/1 -> Fcn/1
  Fcn/1 -> Sum2/1
  Time1/1 -> Sum2/2
  Rate Transition1/1 -> Sum6/1
  MPC Controller/1 -> Rate Transition1/1
  Time8/1 -> Sum6/2
  Unit Delay2/1 -> Sum1/1

== system PVRobusMPC_final/4 x 4 x 4 PV Panel 3/4 x 4 PV Panel 5/4 PV Panel 2/PV Panel 5/Photovolatic Panel ==
  Lambda_UV : Inport
  Lambda_IR : Inport  Port=2
  Tambient : Inport  Port=3
  WS : Inport  Port=4
  PV_Cell_Model : MATLAB Function  TreatAsAtomicUnit=on
  Step Size [sec] : Constant
  Unit Delay : UnitDelay  InitialCondition=Temp_Initial  SampleTime=-1
  Tm_f [K] : Outport
  Pout [Watt] : Outport  Port=2
  Vout [Volts] : Outport  Port=3
  wires:
  PV_Cell_Model/3(VL) -> Vout [Volts]/1
  Step Size [sec]/1 -> PV_Cell_Model/4(Time)
  Lambda_IR/1 -> PV_Cell_Model/3(Lambda_IR)
  Lambda_UV/1 -> PV_Cell_Model/2(Lambda_UV)
  PV_Cell_Model/1(Tm_f) -> Tm_f [K]/1, Unit Delay/1
  Unit Delay/1 -> PV_Cell_Model/1(Tm_i)
  PV_Cell_Model/2(QQ) -> Pout [Watt]/1
  Tambient/1 -> PV_Cell_Model/5(Tambient)
  WS/1 -> PV_Cell_Model/6(WS)

== system PVRobusMPC_final/4 x 4 x 4 PV Panel 3/4 x 4 PV Panel 5/4 PV Panel 2/PV Panel 6/PV MPC ==
  Tm_f : Inport
  Tambient : Inport  Port=2
  Fcn : Fcn  Expr=0.916 *u(1)+79
  MPC Controller : mpclib/MPC Controller  SCDEnableBlockLinearizationSpecification=on  mpcobj=mpc1  is_multiple=0  enable_value=0  return_u0=off  updateMPCinCallerWorkspace=on  ref_from_ws=off  ref_signal_name=[]  ref_preview=off  md_from_ws=off  md_signal_name=[]  md_preview=off  from_project=off  project_file=MPCtask.mat  md_inport=off  mv_inport=off  cost_outport=off  return_sequence=off  return_qpstatus=off  return_state=off  state_inport=off  lims_inport=off  cc_inport=off  ywt_inport=off  is_designfromscratch=0  uwt_inport=off  duwt_inport=off  rhoeps_inport=off  uref_inport=off  n_ts=10  n_p=10  n_mv=1  n_md=1  n_ud=0  n_mo=1  n_uo=0  BlockDataType=double  SampleTimeInherited=off  switch_inport=off
  Rate Transition1 : RateTransition  OutPortSampleTime=1
  Rate Transition2 : RateTransition  OutPortSampleTime=10
  Rate Transition3 : RateTransition  OutPortSampleTime=10
  Sum1 : Sum  Inputs=|+-
  Sum2 : Sum  Inputs=|+-
  Sum6 : Sum  Inputs=|++
  Time1 : Constant  Value=372.8
  Time3 : Constant  Value=372.8
  Time8 : Constant  Value=300
  Unit Delay2 : UnitDelay  InitialCondition=380  SampleTime=-1
  Lambda_UV : Outport
  wires:
  Unit Delay2/1 -> Sum1/1
  Time8/1 -> Sum6/2
  MPC Controller/1 -> Rate Transition1/1
  Rate Transition1/1 -> Sum6/1
  Time1/1 -> Sum2/2
  Fcn/1 -> Sum2/1
  Tambient/1 -> Fcn/1
  Sum2/1 -> Rate Transition2/1
  Sum1/1 -> Rate Transition3/1
  Rate Transition3/1 -> MPC Controller/1
  Rate Transition2/1 -> MPC Controller/2
  Sum6/1 -> Lambda_UV/1
  Time3/1 -> Sum1/2
  Tm_f/1 -> Unit Delay2/1

== system PVRobusMPC_final/4 x 4 x 4 PV Panel 3/4 x 4 PV Panel 5/4 PV Panel 2/PV Panel 6/Photovolatic Panel ==
  Lambda_UV : Inport
  Lambda_IR : Inport  Port=2
  Tambient : Inport  Port=3
  WS : Inport  Port=4
  PV_Cell_Model : MATLAB Function  TreatAsAtomicUnit=on
  Step Size [sec] : Constant
  Unit Delay : UnitDelay  InitialCondition=Temp_Initial  SampleTime=-1
  Tm_f [K] : Outport
  Pout [Watt] : Outport  Port=2
  Vout [Volts] : Outport  Port=3
  wires:
  WS/1 -> PV_Cell_Model/6(WS)
  Tambient/1 -> PV_Cell_Model/5(Tambient)
  PV_Cell_Model/2(QQ) -> Pout [Watt]/1
  Unit Delay/1 -> PV_Cell_Model/1(Tm_i)
  PV_Cell_Model/1(Tm_f) -> Unit Delay/1, Tm_f [K]/1
  Lambda_UV/1 -> PV_Cell_Model/2(Lambda_UV)
  Lambda_IR/1 -> PV_Cell_Model/3(Lambda_IR)
  Step Size [sec]/1 -> PV_Cell_Model/4(Time)
  PV_Cell_Model/3(VL) -> Vout [Volts]/1

== system PVRobusMPC_final/4 x 4 x 4 PV Panel 3/4 x 4 PV Panel 5/4 PV Panel 2/PV Panel 7/PV MPC ==
  Tm_f : Inport
  Tambient : Inport  Port=2
  Fcn : Fcn  Expr=0.916 *u(1)+79
  MPC Controller : mpclib/MPC Controller  SCDEnableBlockLinearizationSpecification=on  mpcobj=mpc1  is_multiple=0  enable_value=0  return_u0=off  updateMPCinCallerWorkspace=on  ref_from_ws=off  ref_signal_name=[]  ref_preview=off  md_from_ws=off  md_signal_name=[]  md_preview=off  from_project=off  project_file=MPCtask.mat  md_inport=off  mv_inport=off  cost_outport=off  return_sequence=off  return_qpstatus=off  return_state=off  state_inport=off  lims_inport=off  cc_inport=off  ywt_inport=off  is_designfromscratch=0  uwt_inport=off  duwt_inport=off  rhoeps_inport=off  uref_inport=off  n_ts=10  n_p=10  n_mv=1  n_md=1  n_ud=0  n_mo=1  n_uo=0  BlockDataType=double  SampleTimeInherited=off  switch_inport=off
  Rate Transition1 : RateTransition  OutPortSampleTime=1
  Rate Transition2 : RateTransition  OutPortSampleTime=10
  Rate Transition3 : RateTransition  OutPortSampleTime=10
  Sum1 : Sum  Inputs=|+-
  Sum2 : Sum  Inputs=|+-
  Sum6 : Sum  Inputs=|++
  Time1 : Constant  Value=372.8
  Time3 : Constant  Value=372.8
  Time8 : Constant  Value=300
  Unit Delay2 : UnitDelay  InitialCondition=380  SampleTime=-1
  Lambda_UV : Outport
  wires:
  Tm_f/1 -> Unit Delay2/1
  Time3/1 -> Sum1/2
  Sum6/1 -> Lambda_UV/1
  Rate Transition2/1 -> MPC Controller/2
  Rate Transition3/1 -> MPC Controller/1
  Sum1/1 -> Rate Transition3/1
  Sum2/1 -> Rate Transition2/1
  Tambient/1 -> Fcn/1
  Fcn/1 -> Sum2/1
  Time1/1 -> Sum2/2
  Rate Transition1/1 -> Sum6/1
  MPC Controller/1 -> Rate Transition1/1
  Time8/1 -> Sum6/2
  Unit Delay2/1 -> Sum1/1

== system PVRobusMPC_final/4 x 4 x 4 PV Panel 3/4 x 4 PV Panel 5/4 PV Panel 2/PV Panel 7/Photovolatic Panel ==
  Lambda_UV : Inport
  Lambda_IR : Inport  Port=2
  Tambient : Inport  Port=3
  WS : Inport  Port=4
  PV_Cell_Model : MATLAB Function  TreatAsAtomicUnit=on
  Step Size [sec] : Constant
  Unit Delay : UnitDelay  InitialCondition=Temp_Initial  SampleTime=-1
  Tm_f [K] : Outport
  Pout [Watt] : Outport  Port=2
  Vout [Volts] : Outport  Port=3
  wires:
  PV_Cell_Model/3(VL) -> Vout [Volts]/1
  Step Size [sec]/1 -> PV_Cell_Model/4(Time)
  Lambda_IR/1 -> PV_Cell_Model/3(Lambda_IR)
  Lambda_UV/1 -> PV_Cell_Model/2(Lambda_UV)
  PV_Cell_Model/1(Tm_f) -> Tm_f [K]/1, Unit Delay/1
  Unit Delay/1 -> PV_Cell_Model/1(Tm_i)
  PV_Cell_Model/2(QQ) -> Pout [Watt]/1
  Tambient/1 -> PV_Cell_Model/5(Tambient)
  WS/1 -> PV_Cell_Model/6(WS)

== system PVRobusMPC_final/4 x 4 x 4 PV Panel 3/4 x 4 PV Panel 5/4 PV Panel 2/PV Panel 8/PV MPC ==
  Tm_f : Inport
  Tambient : Inport  Port=2
  Fcn : Fcn  Expr=0.916 *u(1)+79
  MPC Controller : mpclib/MPC Controller  SCDEnableBlockLinearizationSpecification=on  mpcobj=mpc1  is_multiple=0  enable_value=0  return_u0=off  updateMPCinCallerWorkspace=on  ref_from_ws=off  ref_signal_name=[]  ref_preview=off  md_from_ws=off  md_signal_name=[]  md_preview=off  from_project=off  project_file=MPCtask.mat  md_inport=off  mv_inport=off  cost_outport=off  return_sequence=off  return_qpstatus=off  return_state=off  state_inport=off  lims_inport=off  cc_inport=off  ywt_inport=off  is_designfromscratch=0  uwt_inport=off  duwt_inport=off  rhoeps_inport=off  uref_inport=off  n_ts=10  n_p=10  n_mv=1  n_md=1  n_ud=0  n_mo=1  n_uo=0  BlockDataType=double  SampleTimeInherited=off  switch_inport=off
  Rate Transition1 : RateTransition  OutPortSampleTime=1
  Rate Transition2 : RateTransition  OutPortSampleTime=10
  Rate Transition3 : RateTransition  OutPortSampleTime=10
  Sum1 : Sum  Inputs=|+-
  Sum2 : Sum  Inputs=|+-
  Sum6 : Sum  Inputs=|++
  Time1 : Constant  Value=372.8
  Time3 : Constant  Value=372.8
  Time8 : Constant  Value=300
  Unit Delay2 : UnitDelay  InitialCondition=380  SampleTime=-1
  Lambda_UV : Outport
  wires:
  Unit Delay2/1 -> Sum1/1
  Time8/1 -> Sum6/2
  MPC Controller/1 -> Rate Transition1/1
  Rate Transition1/1 -> Sum6/1
  Time1/1 -> Sum2/2
  Fcn/1 -> Sum2/1
  Tambient/1 -> Fcn/1
  Sum2/1 -> Rate Transition2/1
  Sum1/1 -> Rate Transition3/1
  Rate Transition3/1 -> MPC Controller/1
  Rate Transition2/1 -> MPC Controller/2
  Sum6/1 -> Lambda_UV/1
  Time3/1 -> Sum1/2
  Tm_f/1 -> Unit Delay2/1

== system PVRobusMPC_final/4 x 4 x 4 PV Panel 3/4 x 4 PV Panel 5/4 PV Panel 2/PV Panel 8/Photovolatic Panel ==
  Lambda_UV : Inport
  Lambda_IR : Inport  Port=2
  Tambient : Inport  Port=3
  WS : Inport  Port=4
  PV_Cell_Model : MATLAB Function  TreatAsAtomicUnit=on
  Step Size [sec] : Constant
  Unit Delay : UnitDelay  InitialCondition=Temp_Initial  SampleTime=-1
  Tm_f [K] : Outport
  Pout [Watt] : Outport  Port=2
  Vout [Volts] : Outport  Port=3
  wires:
  WS/1 -> PV_Cell_Model/6(WS)
  Tambient/1 -> PV_Cell_Model/5(Tambient)
  PV_Cell_Model/2(QQ) -> Pout [Watt]/1
  Unit Delay/1 -> PV_Cell_Model/1(Tm_i)
  PV_Cell_Model/1(Tm_f) -> Unit Delay/1, Tm_f [K]/1
  Lambda_UV/1 -> PV_Cell_Model/2(Lambda_UV)
  Lambda_IR/1 -> PV_Cell_Model/3(Lambda_IR)
  Step Size [sec]/1 -> PV_Cell_Model/4(Time)
  PV_Cell_Model/3(VL) -> Vout [Volts]/1

== system PVRobusMPC_final/4 x 4 x 4 PV Panel 3/4 x 4 PV Panel 5/4 PV Panel 3/PV Panel 5/PV MPC ==
  Tm_f : Inport
  Tambient : Inport  Port=2
  Fcn : Fcn  Expr=0.916 *u(1)+79
  MPC Controller : mpclib/MPC Controller  SCDEnableBlockLinearizationSpecification=on  mpcobj=mpc1  is_multiple=0  enable_value=0  return_u0=off  updateMPCinCallerWorkspace=on  ref_from_ws=off  ref_signal_name=[]  ref_preview=off  md_from_ws=off  md_signal_name=[]  md_preview=off  from_project=off  project_file=MPCtask.mat  md_inport=off  mv_inport=off  cost_outport=off  return_sequence=off  return_qpstatus=off  return_state=off  state_inport=off  lims_inport=off  cc_inport=off  ywt_inport=off  is_designfromscratch=0  uwt_inport=off  duwt_inport=off  rhoeps_inport=off  uref_inport=off  n_ts=10  n_p=10  n_mv=1  n_md=1  n_ud=0  n_mo=1  n_uo=0  BlockDataType=double  SampleTimeInherited=off  switch_inport=off
  Rate Transition1 : RateTransition  OutPortSampleTime=1
  Rate Transition2 : RateTransition  OutPortSampleTime=10
  Rate Transition3 : RateTransition  OutPortSampleTime=10
  Sum1 : Sum  Inputs=|+-
  Sum2 : Sum  Inputs=|+-
  Sum6 : Sum  Inputs=|++
  Time1 : Constant  Value=372.8
  Time3 : Constant  Value=372.8
  Time8 : Constant  Value=300
  Unit Delay2 : UnitDelay  InitialCondition=380  SampleTime=-1
  Lambda_UV : Outport
  wires:
  Unit Delay2/1 -> Sum1/1
  Time8/1 -> Sum6/2
  MPC Controller/1 -> Rate Transition1/1
  Rate Transition1/1 -> Sum6/1
  Time1/1 -> Sum2/2
  Fcn/1 -> Sum2/1
  Tambient/1 -> Fcn/1
  Sum2/1 -> Rate Transition2/1
  Sum1/1 -> Rate Transition3/1
  Rate Transition3/1 -> MPC Controller/1
  Rate Transition2/1 -> MPC Controller/2
  Sum6/1 -> Lambda_UV/1
  Time3/1 -> Sum1/2
  Tm_f/1 -> Unit Delay2/1

== system PVRobusMPC_final/4 x 4 x 4 PV Panel 3/4 x 4 PV Panel 5/4 PV Panel 3/PV Panel 5/Photovolatic Panel ==
  Lambda_UV : Inport
  Lambda_IR : Inport  Port=2
  Tambient : Inport  Port=3
  WS : Inport  Port=4
  PV_Cell_Model : MATLAB Function  TreatAsAtomicUnit=on
  Step Size [sec] : Constant
  Unit Delay : UnitDelay  InitialCondition=Temp_Initial  SampleTime=-1
  Tm_f [K] : Outport
  Pout [Watt] : Outport  Port=2
  Vout [Volts] : Outport  Port=3
  wires:
  WS/1 -> PV_Cell_Model/6(WS)
  Tambient/1 -> PV_Cell_Model/5(Tambient)
  PV_Cell_Model/2(QQ) -> Pout [Watt]/1
  Unit Delay/1 -> PV_Cell_Model/1(Tm_i)
  PV_Cell_Model/1(Tm_f) -> Unit Delay/1, Tm_f [K]/1
  Lambda_UV/1 -> PV_Cell_Model/2(Lambda_UV)
  Lambda_IR/1 -> PV_Cell_Model/3(Lambda_IR)
  Step Size [sec]/1 -> PV_Cell_Model/4(Time)
  PV_Cell_Model/3(VL) -> Vout [Volts]/1

== system PVRobusMPC_final/4 x 4 x 4 PV Panel 3/4 x 4 PV Panel 5/4 PV Panel 3/PV Panel 6/PV MPC ==
  Tm_f : Inport
  Tambient : Inport  Port=2
  Fcn : Fcn  Expr=0.916 *u(1)+79
  MPC Controller : mpclib/MPC Controller  SCDEnableBlockLinearizationSpecification=on  mpcobj=mpc1  is_multiple=0  enable_value=0  return_u0=off  updateMPCinCallerWorkspace=on  ref_from_ws=off  ref_signal_name=[]  ref_preview=off  md_from_ws=off  md_signal_name=[]  md_preview=off  from_project=off  project_file=MPCtask.mat  md_inport=off  mv_inport=off  cost_outport=off  return_sequence=off  return_qpstatus=off  return_state=off  state_inport=off  lims_inport=off  cc_inport=off  ywt_inport=off  is_designfromscratch=0  uwt_inport=off  duwt_inport=off  rhoeps_inport=off  uref_inport=off  n_ts=10  n_p=10  n_mv=1  n_md=1  n_ud=0  n_mo=1  n_uo=0  BlockDataType=double  SampleTimeInherited=off  switch_inport=off
  Rate Transition1 : RateTransition  OutPortSampleTime=1
  Rate Transition2 : RateTransition  OutPortSampleTime=10
  Rate Transition3 : RateTransition  OutPortSampleTime=10
  Sum1 : Sum  Inputs=|+-
  Sum2 : Sum  Inputs=|+-
  Sum6 : Sum  Inputs=|++
  Time1 : Constant  Value=372.8
  Time3 : Constant  Value=372.8
  Time8 : Constant  Value=300
  Unit Delay2 : UnitDelay  InitialCondition=380  SampleTime=-1
  Lambda_UV : Outport
  wires:
  Tm_f/1 -> Unit Delay2/1
  Time3/1 -> Sum1/2
  Sum6/1 -> Lambda_UV/1
  Rate Transition2/1 -> MPC Controller/2
  Rate Transition3/1 -> MPC Controller/1
  Sum1/1 -> Rate Transition3/1
  Sum2/1 -> Rate Transition2/1
  Tambient/1 -> Fcn/1
  Fcn/1 -> Sum2/1
  Time1/1 -> Sum2/2
  Rate Transition1/1 -> Sum6/1
  MPC Controller/1 -> Rate Transition1/1
  Time8/1 -> Sum6/2
  Unit Delay2/1 -> Sum1/1

== system PVRobusMPC_final/4 x 4 x 4 PV Panel 3/4 x 4 PV Panel 5/4 PV Panel 3/PV Panel 6/Photovolatic Panel ==
  Lambda_UV : Inport
  Lambda_IR : Inport  Port=2
  Tambient : Inport  Port=3
  WS : Inport  Port=4
  PV_Cell_Model : MATLAB Function  TreatAsAtomicUnit=on
  Step Size [sec] : Constant
  Unit Delay : UnitDelay  InitialCondition=Temp_Initial  SampleTime=-1
  Tm_f [K] : Outport
  Pout [Watt] : Outport  Port=2
  Vout [Volts] : Outport  Port=3
  wires:
  PV_Cell_Model/3(VL) -> Vout [Volts]/1
  Step Size [sec]/1 -> PV_Cell_Model/4(Time)
  Lambda_IR/1 -> PV_Cell_Model/3(Lambda_IR)
  Lambda_UV/1 -> PV_Cell_Model/2(Lambda_UV)
  PV_Cell_Model/1(Tm_f) -> Tm_f [K]/1, Unit Delay/1
  Unit Delay/1 -> PV_Cell_Model/1(Tm_i)
  PV_Cell_Model/2(QQ) -> Pout [Watt]/1
  Tambient/1 -> PV_Cell_Model/5(Tambient)
  WS/1 -> PV_Cell_Model/6(WS)
